simulink model "synthesis_snh"  (R2020a)
settings: Solver=FixedStepAuto  StartTime=0.0  StopTime=inf  FixedStep=0.05  RelTol=1e-3
libraries: robotlib x12, dspsigops x1
settings Model: Creator=ivory  LastModifiedBy=ivory
settings OptimizationCC: EnhancedBackFolding=on  PassReuseOutputArgsAs=Individual arguments  ZeroExternalMemoryAtStartup=off  ZeroInternalMemoryAtStartup=off  MaxStackSize=64  OptimizeBlockOrder=speed  DifferentSizesBufferReuse=on  OptimizationCustomize=off  EfficientTunableParamExpr=on
settings DebuggingCC: ParameterTunabilityLossMsg=error
settings HardwareCC: ProdBitPerPointer=32  ProdBitPerSizeT=32  ProdBitPerPtrDiffT=32  ProdLargestAtomicFloat=None  ProdIntDivRoundTo=Undefined  ProdEndianess=Unspecified  ProdWordSize=32  ProdHWDeviceType=Generic->Unspecified (assume 32-bit Generic)
settings SFSimCC: MATLABDynamicMemAlloc=off
settings RTWCC: SystemTargetFile=ert.tlc  HardwareBoard=Robot Operating System (ROS)  TemplateMakefile=ert_default_tmf  Toolchain=Catkin  TargetLang=C++
settings CodeAppCC: ForceParamTrailComments=on  IgnoreCustomStorageClasses=off  OperatorAnnotations=on  SimulinkDataObjDesc=on  SFDataObjDesc=on  InsertBlockDesc=on
settings ERTTargetCC: SupportContinuousTime=on

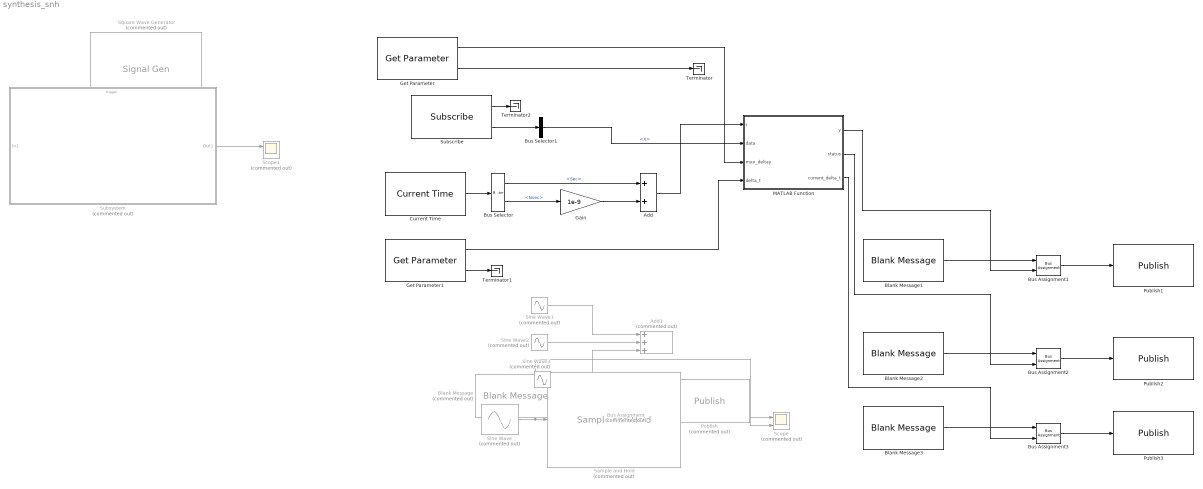
== system synthesis_snh ==
  Add : Sum
  Add1 : Sum  Commented=on  Inputs=+++
  Blank Message : robotlib/Blank Message  Commented=on  messageClass=Message  entityType=std_msgs/Float64  messageType=std_msgs/Float64  SampleTime=inf
  Blank Message1 : robotlib/Blank Message  messageClass=Message  entityType=geometry_msgs/Twist  messageType=geometry_msgs/Twist  SampleTime=inf
  Blank Message2 : robotlib/Blank Message  messageClass=Message  entityType=std_msgs/Float64  messageType=std_msgs/Float64  SampleTime=inf
  Blank Message3 : robotlib/Blank Message  messageClass=Message  entityType=std_msgs/Float64  messageType=std_msgs/Float64  SampleTime=inf
  Bus Assignment : BusAssignment  Commented=on  AssignedSignals=Data
  Bus Assignment1 : BusAssignment  AssignedSignals=Linear.X
  Bus Assignment2 : BusAssignment  AssignedSignals=Data
  Bus Assignment3 : BusAssignment  AssignedSignals=Data
  Bus Selector : BusSelector  OutputSignals=Sec,Nsec
  Bus Selector1 : BusSelector  OutputSignals=Linear.X
  Current Time : robotlib/Current Time  OutputFormat=bus  SampleTime=-1  ModelName=synthesis_snh
      settings: SourceProductBaseCode=RR
  Gain : Gain  Gain=1e-9
  Get Parameter : robotlib/Get Parameter  ParameterSource=Specify your own  ParameterName=max_deltay  ParameterType=double  ParameterMaxArrayLength=16  ParameterInitialValue=1.0  SampleTime=-1  ShowErrorCodeOutput=on  ModelName=synthesis_snh  BlockId=ParamGet_synthesis_snh_17
      settings: SourceProductBaseCode=RR
  Get Parameter1 : robotlib/Get Parameter  ParameterSource=Specify your own  ParameterName=delta_t  ParameterType=double  ParameterMaxArrayLength=16  ParameterInitialValue=1.0  SampleTime=-1  ShowErrorCodeOutput=on  ModelName=synthesis_snh  BlockId=ParamGet_synthesis_snh_18
      settings: SourceProductBaseCode=RR
  MATLAB Function : MATLAB Function  TreatAsAtomicUnit=on
  Publish : robotlib/Publish  Commented=on  topicSource=Specify your own  topic=input  messageType=std_msgs/Float64  messageQueueLength=1
  Publish1 : robotlib/Publish  topicSource=Specify your own  topic=output  messageType=geometry_msgs/Twist  messageQueueLength=1
  Publish2 : robotlib/Publish  topicSource=Specify your own  topic=status  messageType=std_msgs/Float64  messageQueueLength=1
  Publish3 : robotlib/Publish  topicSource=Specify your own  topic=current_delta_t  messageType=std_msgs/Float64  messageQueueLength=1
  Sample and Hold : dspsigops/Sample and Hold  Commented=on  trig=Rising edge  initCond=0  latchinput=off
  Scope : Scope  Commented=on  NumInputPorts=2
  Scope1 : Scope  Commented=on  NumInputPorts=2
  Sine Wave : Sin  Commented=on  Amplitude=22  Bias=6  SampleTime=0
  Sine Wave1 : Sin  Commented=on  Amplitude=6  SampleTime=0
  Sine Wave2 : Sin  Commented=on  Amplitude=9.3  Bias=3.2  Frequency=0.244  Phase=4  SampleTime=0
  Sine Wave3 : Sin  Commented=on  Bias=9  Frequency=0.01  Phase=3  SampleTime=0
  Square Wave Generator : SignalGenerator  Commented=on  WaveForm=square  TimeSource=Use external signal  Frequency=1/1.2
  Subscribe : robotlib/Subscribe  topicSource=Specify your own  topic=cmd_vel  messageType=geometry_msgs/Twist  sampleTime=-1  messageQueueLength=1
  Subsystem : Subsystem  Commented=on
  Terminator : Terminator
  Terminator1 : Terminator
  Terminator2 : Terminator
  wires:
  Current Time/1 -> Bus Selector/1
  Bus Selector/2 -> Gain/1  "<Nsec>"
  Bus Selector/1 -> Add/1  "<Sec>"
  Gain/1 -> Add/2
  Sine Wave/1 -> Scope/2, Sample and Hold/1
  Sample and Hold/1 -> Scope/1
  Get Parameter1/2 -> Terminator1/1
  Subsystem/1(Out1) -> Scope1/1
  Sine Wave2/1 -> Add1/2
  Sine Wave3/1 -> Add1/3
  Sine Wave1/1 -> Add1/1
  Get Parameter/2 -> Terminator/1
  Get Parameter/1 -> MATLAB Function/3(max_deltay)
  Get Parameter1/1 -> MATLAB Function/4(delta_t)
  Add/1 -> MATLAB Function/1(t)
  Bus Assignment/1 -> Publish/1
  Blank Message/1 -> Bus Assignment/1
  MATLAB Function/1(y) -> Bus Assignment1/2
  Bus Assignment1/1 -> Publish1/1
  Blank Message1/1 -> Bus Assignment1/1
  Blank Message2/1 -> Bus Assignment2/1
  Bus Assignment2/1 -> Publish2/1
  MATLAB Function/2(status) -> Bus Assignment2/2
  MATLAB Function/3(current_delta_t) -> Bus Assignment3/2
  Bus Assignment3/1 -> Publish3/1
  Blank Message3/1 -> Bus Assignment3/1
  Subscribe/1 -> Terminator2/1
  Subscribe/2 -> Bus Selector1/1
  Bus Selector1/1 -> MATLAB Function/2(data)  "<X>"

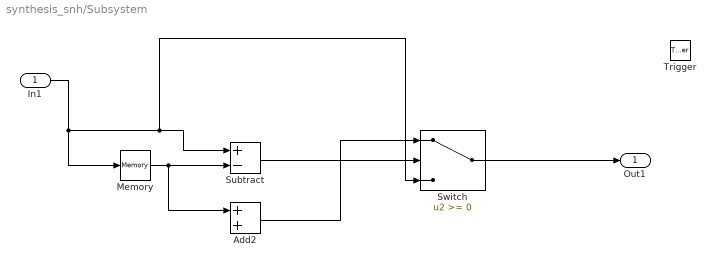
== system synthesis_snh/Subsystem ==
  In1 : Inport
  Trigger : TriggerPort  VariantControl=Variant  PortDimensions=1
  Add2 : Sum
  Memory : Memory  InheritSampleTime=on
  Subtract : Sum  Inputs=+-
  Switch : Switch
  Out1 : Outport
  wires:
  Memory/1 -> Add2/1, Subtract/2
  Switch/1 -> Out1/1
  Add2/1 -> Switch/1
  In1/1 -> Memory/1, Switch/3, Subtract/1
  Subtract/1 -> Switch/2

== matlab function synthesis_snh/MATLAB Function ==
  data: t input; y output; data input; max_deltay input; delta_t input; status output; current_delta_t output
function [y, status, current_delta_t] = fcn(t, data, max_deltay, delta_t)

persistent last_time
persistent last_value

if isempty(last_time)
    last_time = t;
    last_value = data;
    y= data;
    status = -1;
    current_delta_t = 0;
else
    
    current_delta_t = t - last_time;
    if (t - last_time <= delta_t)
        
        
        y = last_value;
        status = 0;
    else
        if( abs(data - last_value) >= max_deltay)

            y = last_value + max_deltay*sign(data - last_value);
            last_value = y;
            status = 1;
        else
            y = data;
            last_value = data;
            status = 2;
        end
        last_time = t;
    end

end


 
end
